simulink library "Sources_lib"  (R2023a)
settings: Solver=VariableStepAuto  StartTime=0.0  StopTime=10.0  RelTol=1e-3
values from neighbouring files (symbols this model uses):
  f_si = 50    [controlvsource.m]
  max_f_dev_si = 0.5    [controlvsource.m]
  phi_init = 0    [controlvsource.m]
  rocof_des_si = 1    [controlvsource.m]
  t_rocof = 0.5    [controlvsource.m]
  v_rms_ln_si = 230    [controlvsource.m]
undefined symbols (not defined in the file or in its folder): DiscIntNeverNeededParam
libraries: ee_lib x1, fl_lib x1, eeTransforms x1, nesl_utility x1
settings Model: Creator=e2n051  LastModifiedBy=e2n051

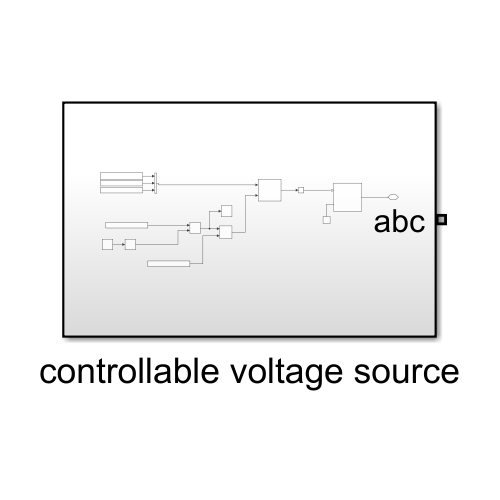
[thumbnail: Simulink's stored preview of the top-level diagram]
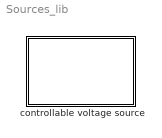
== system Sources_lib ==
  controllable voltage source : Subsystem

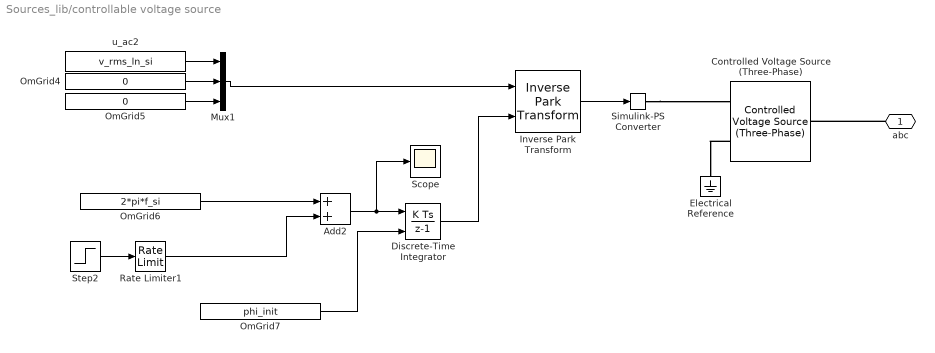
== system Sources_lib/controllable voltage source ==
  Add2 : Sum
  Controlled Voltage Source (Three-Phase) : ee_lib/Sources/Controlled Voltage Source (Three-Phase)  input_option=ee.enum.inputType.instantaneous  FRated=60 Hz
      settings: InternalSimscapePortConfiguration="{\"Bottom\":[],\"Left\":[{\"id\":\"S\",\"label\":\"S\",\"type\":\"input\"},{\"id\":\"n\",\"label\":\"n\",\"type\":\"foundation.electrical.electrical\"}],\"Right\":[{\"id\":\"N\",\"label\":\"~\",\"type\":\"foundation.electrical.three_phase\"}],\"Top\":[]}"
  Discrete-Time Integrator : DiscreteIntegrator  InitialConditionSource=external  SampleTime=-1  ICPrevOutput=DiscIntNeverNeededParam  ICPrevScaledInput=DiscIntNeverNeededParam
  Electrical Reference : fl_lib/Electrical/Electrical Elements/Electrical Reference
  Inverse Park Transform : eeTransforms/Inverse Park Transform  AxisAlignment=Q-axis  PowerInvariant=off
      settings: LibrarySourceBlock=|
      | ee_sl_lib/Mathematical
      | Transforms/Inverse
      | Park Transform
  Mux1 : Mux  Inputs=3
  OmGrid4 : Constant  Value=0
  OmGrid5 : Constant  Value=0
  OmGrid6 : Constant  Value=2*pi*f_si
  OmGrid7 : Constant  Value=phi_init
  Rate Limiter1 : RateLimiter  RisingSlewLimit=2*pi*rocof_des_si  FallingSlewLimit=-2*pi*rocof_des_si  SampleTimeMode=inherited
  Scope : Scope
  Simulink-PS Converter : nesl_utility/Simulink-PS Converter  PhysicalDomain=network_engine_domain  SubClassName=ps_input  LeftPortType=input  RightPortType=output  PseudoPeriodic=off  Frequencies=[]  NoiseDistribution=none  NoiseParameters=[]  Unit=1  AffineConversion=off  FilteringAndDerivatives=provide  SimscapeFilterOrder=1  InputFilterTimeConstant=0.001  UdotUserProvided=0
  Step2 : Step  Time=t_rocof  After=2*pi*max_f_dev_si  SampleTime=0
  u_ac2 : Constant  Value=v_rms_ln_si
  abc : PMIOPort  Side=Right
  wires:
  OmGrid5/1 -> Mux1/3
  Mux1/1 -> Inverse Park Transform/1
  u_ac2/1 -> Mux1/1
  OmGrid4/1 -> Mux1/2
  Inverse Park Transform/1 -> Simulink-PS Converter/1
  Discrete-Time Integrator/1 -> Inverse Park Transform/2
  OmGrid7/1 -> Discrete-Time Integrator/2
  Step2/1 -> Rate Limiter1/1
  OmGrid6/1 -> Add2/1
  Add2/1 -> Scope/1, Discrete-Time Integrator/1
  Rate Limiter1/1 -> Add2/2
  connections:
  Simulink-PS Converter/RConn1 -- Controlled Voltage Source (Three-Phase)/LConn1
  Controlled Voltage Source (Three-Phase)/LConn2 -- Electrical Reference/LConn1
  abc/RConn1 -- Controlled Voltage Source (Three-Phase)/RConn1
